simulink model "Buck_Due"  (R2020a)
settings: Solver=FixedStepAuto  StartTime=0.0  StopTime=10  FixedStep=T  RelTol=1e-3  EnableMultiTasking=on
undefined symbols (not defined in the file): C, Ki_IL, Kp_IL, Kp_Uc, L, rL, T, Ubat
libraries: arduinolib x12, simulink x8, powerlib_meascontrol x1
settings Model: SILPILModeSetting=veronly  ExtModeTrigDuration=2  Creator=Nguyen Tung  LastModifiedBy=Nguyen Tung
settings OptimizationCC: StrengthReduction=on  PassReuseOutputArgsAs=Individual arguments  ZeroExternalMemoryAtStartup=off  ZeroInternalMemoryAtStartup=off  MaxStackSize=64  OptimizeBlockOrder=speed  OptimizationPriority=Speed  OptimizationCustomize=off  MultiThreadedLoops=on  EfficientTunableParamExpr=on
settings DebuggingCC: ParameterTunabilityLossMsg=error
settings HardwareCC: ProdBitPerPointer=32  ProdBitPerSizeT=32  ProdBitPerPtrDiffT=32  ProdLargestAtomicInteger=Long  ProdLargestAtomicFloat=Double  ProdWordSize=32  ProdHWDeviceType=ARM Compatible->ARM Cortex
settings SFSimCC: MATLABDynamicMemAlloc=off
settings RTWCC: SystemTargetFile=ert.tlc  HardwareBoard=Arduino Due  TLCOptions=-aInlineSetEventsForThisBaseRateFcn=TLC_FALSE -aSuppressMultiTaskScheduler=TLC_FALSE -aRateBasedStepFcn=1  TemplateMakefile=ert_default_tmf  Toolchain=Arduino ARM  BuildConfiguration=Faster Runs
settings CodeAppCC: ForceParamTrailComments=on  IgnoreCustomStorageClasses=off  OperatorAnnotations=on  SimulinkDataObjDesc=on  SFDataObjDesc=on  InsertBlockDesc=on
settings ERTTargetCC: SupportContinuousTime=on  SupportVariableSizeSignals=on  ExtModeStaticAllocSize=10000

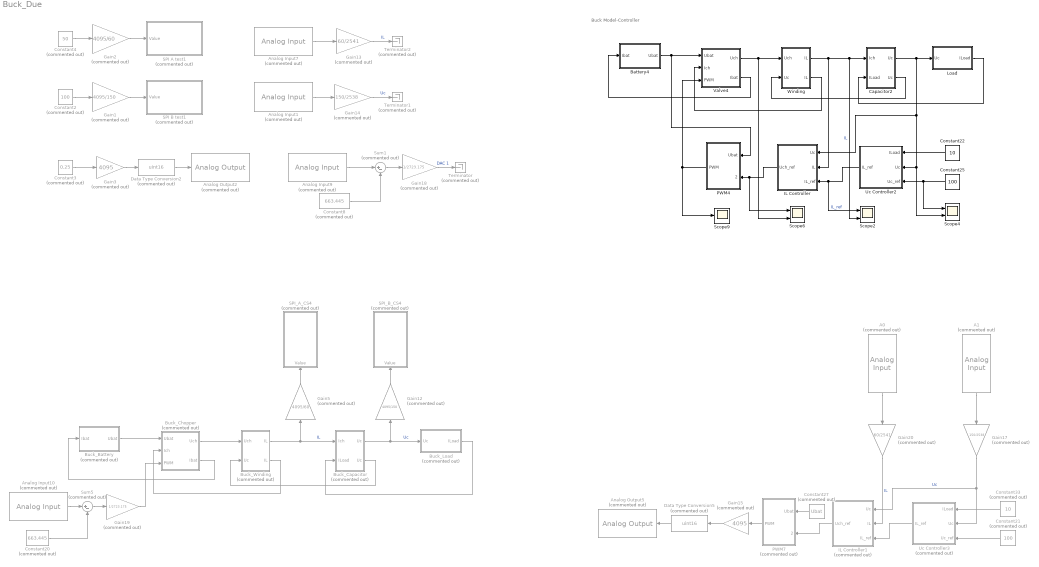
== system Buck_Due ==
  note: Buck Model-Controller
  A0 : arduinolib/Analog Input  Commented=on  pinNumber=0  ReadResultsOnly=off  ConversionTriggerSource=Software  ExternalTriggerType=uint32( 0 )  OutputDataType=uint16  EnableConversionCompleteNotify=off  EnableOuputStatus=off  SampleTime=T  blockPlatform=arduino
  A1 : arduinolib/Analog Input  Commented=on  pinNumber=1  ReadResultsOnly=off  ConversionTriggerSource=Software  ExternalTriggerType=uint32( 0 )  OutputDataType=uint16  EnableConversionCompleteNotify=off  EnableOuputStatus=off  SampleTime=T  blockPlatform=arduino
  Analog Input1 : arduinolib/Analog Input  Commented=on  pinNumber=1  ReadResultsOnly=off  ConversionTriggerSource=Software  ExternalTriggerType=uint32( 0 )  OutputDataType=uint16  EnableConversionCompleteNotify=off  EnableOuputStatus=off  SampleTime=T  blockPlatform=arduino
  Analog Input10 : arduinolib/Analog Input  Commented=on  pinNumber=1  ReadResultsOnly=off  ConversionTriggerSource=Software  ExternalTriggerType=uint32( 0 )  OutputDataType=uint16  EnableConversionCompleteNotify=off  EnableOuputStatus=off  SampleTime=T  blockPlatform=arduino
  Analog Input7 : arduinolib/Analog Input  Commented=on  pinNumber=0  ReadResultsOnly=off  ConversionTriggerSource=Software  ExternalTriggerType=uint32( 0 )  OutputDataType=uint16  EnableConversionCompleteNotify=off  EnableOuputStatus=off  SampleTime=T  blockPlatform=arduino
  Analog Input9 : arduinolib/Analog Input  Commented=on  pinNumber=1  ReadResultsOnly=off  ConversionTriggerSource=Software  ExternalTriggerType=uint32( 0 )  OutputDataType=uint16  EnableConversionCompleteNotify=off  EnableOuputStatus=off  SampleTime=T  blockPlatform=arduino
  Analog Output2 : arduinolib/Analog Output  Commented=on  DACpin=DAC1  blockPlatform=arduino
      settings: SourceProductBaseCode=ARDUINO
  Analog Output5 : arduinolib/Analog Output  Commented=on  DACpin=DAC1  blockPlatform=arduino
      settings: SourceProductBaseCode=ARDUINO
  Battery4 : Subsystem  AncestorBlock=simulink/REM/SE
      mask Display:
      | plot(0,0,100,100, 1.2*[50,57.68,60.77,63.08,64.97,66.58,68,69.26,70.4, 	71.42,72.36,78.28,80,78.28,72.36,71.42,70.4, 	69.26,68,66.58,64.97,63.08,60.77,57.68,50,42.32, 	39.23,36.92,35.03,33.42,32,30.74,29.6,28.58, 	27.64,21.72,20,21.72,27.64,28.58,29.6,30.74,32, 	33.42,35.03,36.92,39.23,42.32,50]-10, 1.2*[20,21,22,23,24,25,26,27,28,29,30,40,50,60,70,71,72, 	73,74,75,76,77,78,79,80,79,78,77,76,75,74,73,72, 	71,70,60,50,40,30,29,28,27,26,25,24,23,22,21,20]-10)
      | disp('ES')
  Buck_Battery : Subsystem  Commented=on  AncestorBlock=simulink/REM/SE
      mask Display:
      | plot(0,0,100,100, 1.2*[50,57.68,60.77,63.08,64.97,66.58,68,69.26,70.4, 	71.42,72.36,78.28,80,78.28,72.36,71.42,70.4, 	69.26,68,66.58,64.97,63.08,60.77,57.68,50,42.32, 	39.23,36.92,35.03,33.42,32,30.74,29.6,28.58, 	27.64,21.72,20,21.72,27.64,28.58,29.6,30.74,32, 	33.42,35.03,36.92,39.23,42.32,50]-10, 1.2*[20,21,22,23,24,25,26,27,28,29,30,40,50,60,70,71,72, 	73,74,75,76,77,78,79,80,79,78,77,76,75,74,73,72, 	71,70,60,50,40,30,29,28,27,26,25,24,23,22,21,20]-10)
      | disp('ES')
  Buck_Capacitor : Subsystem  Commented=on  AncestorBlock=simulink/REM/EA  mask(CM){}
      mask Display: plot(0,0,100,100,[10,10,90,90,10],[90,10,10,90,90], [10,90],[10,90])
  Buck_Chopper : Subsystem  Commented=on  AncestorBlock=simulink/REM/EC Elec  mask(Hacheur){}
      mask Display: plot(0,0,100,100,[10,10,90,90,10],[90,10,10,90,90])
  Buck_Load : Subsystem  Commented=on  AncestorBlock=simulink/REM/SE
      mask Display:
      | plot(0,0,100,100, 1.2*[50,57.68,60.77,63.08,64.97,66.58,68,69.26,70.4, 	71.42,72.36,78.28,80,78.28,72.36,71.42,70.4, 	69.26,68,66.58,64.97,63.08,60.77,57.68,50,42.32, 	39.23,36.92,35.03,33.42,32,30.74,29.6,28.58, 	27.64,21.72,20,21.72,27.64,28.58,29.6,30.74,32, 	33.42,35.03,36.92,39.23,42.32,50]-10, 1.2*[20,21,22,23,24,25,26,27,28,29,30,40,50,60,70,71,72, 	73,74,75,76,77,78,79,80,79,78,77,76,75,74,73,72, 	71,70,60,50,40,30,29,28,27,26,25,24,23,22,21,20]-10)
      | disp('MS')
  Buck_Winding : Subsystem  Commented=on  AncestorBlock=simulink/REM/EA  mask(CM){}
      mask Display: plot(0,0,100,100,[10,10,90,90,10],[90,10,10,90,90], [10,90],[10,90])
  Capacitor2 : Subsystem  AncestorBlock=simulink/REM/EA  mask(CM){}
      mask Display: plot(0,0,100,100,[10,10,90,90,10],[90,10,10,90,90], [10,90],[10,90])
  Constant2 : Constant  Commented=on  Value=100
  Constant20 : Constant  Commented=on  Value=663.445
  Constant21 : Constant  Commented=on  Value=100
  Constant22 : Constant  Value=10
  Constant25 : Constant  Value=100  SampleTime=T
  Constant27 : Constant  Commented=on  Value=Ubat
  Constant3 : Constant  Commented=on  Value=0.25
  Constant33 : Constant  Commented=on  Value=10
  Constant4 : Constant  Commented=on  Value=50
  Constant8 : Constant  Commented=on  Value=663.445
  Data Type Conversion2 : DataTypeConversion  Commented=on  OutDataTypeStr=uint16  RndMeth=Nearest
  Data Type Conversion5 : DataTypeConversion  Commented=on  OutDataTypeStr=uint16  RndMeth=Nearest
  Gain1 : Gain  Commented=on  Gain=4095/150
  Gain12 : Gain  Commented=on  Gain=4095/150
  Gain13 : Gain  Commented=on  Gain=60/2541
  Gain14 : Gain  Commented=on  Gain=150/2538
  Gain15 : Gain  Commented=on  Gain=4095
  Gain17 : Gain  Commented=on  Gain=150/2538
  Gain18 : Gain  Commented=on  Gain=1/2723.175
  Gain19 : Gain  Commented=on  Gain=1/2723.175
  Gain2 : Gain  Commented=on  Gain=4095/60
  Gain20 : Gain  Commented=on  Gain=60/2541
  Gain3 : Gain  Commented=on  Gain=4095
  Gain5 : Gain  Commented=on  Gain=4095/60
  IL Controller : Subsystem  AncestorBlock=simulink/SMC/Asservissement Correcteur IP
      mask Display: plot(0,0,100,100, [10,30,90,70,10,90],[90,10,10,90,90,10])
  IL Controller1 : Subsystem  Commented=on  AncestorBlock=simulink/SMC/Asservissement Correcteur IP
      mask Display: plot(0,0,100,100, [10,30,90,70,10,90],[90,10,10,90,90,10])
  Load : Subsystem  AncestorBlock=simulink/REM/SE
      mask Display:
      | plot(0,0,100,100, 1.2*[50,57.68,60.77,63.08,64.97,66.58,68,69.26,70.4, 	71.42,72.36,78.28,80,78.28,72.36,71.42,70.4, 	69.26,68,66.58,64.97,63.08,60.77,57.68,50,42.32, 	39.23,36.92,35.03,33.42,32,30.74,29.6,28.58, 	27.64,21.72,20,21.72,27.64,28.58,29.6,30.74,32, 	33.42,35.03,36.92,39.23,42.32,50]-10, 1.2*[20,21,22,23,24,25,26,27,28,29,30,40,50,60,70,71,72, 	73,74,75,76,77,78,79,80,79,78,77,76,75,74,73,72, 	71,70,60,50,40,30,29,28,27,26,25,24,23,22,21,20]-10)
      | disp('MS')
  PWM4 : Subsystem  AncestorBlock=simulink/SMC/Inversion EC avec mesure
      mask Display: plot(0,0,100,100,[10,30,90,70,10],[90,10,10,90,90])
  PWM7 : Subsystem  Commented=on  AncestorBlock=simulink/SMC/Inversion EC avec mesure
      mask Display: plot(0,0,100,100,[10,30,90,70,10],[90,10,10,90,90])
  SPI A test1 : Subsystem  Commented=on
  SPI B test1 : Subsystem  Commented=on
  SPI_A_CS4 : Subsystem  Commented=on
  SPI_B_CS4 : Subsystem  Commented=on
  Scope2 : Scope  NumInputPorts=2
  Scope4 : Scope  NumInputPorts=2
  Scope6 : Scope  NumInputPorts=2
  Scope9 : Scope
  Sum1 : Sum  Commented=on  Inputs=|+-
  Sum5 : Sum  Commented=on  Inputs=|+-
  Terminator : Terminator  Commented=on
  Terminator1 : Terminator  Commented=on
  Terminator2 : Terminator  Commented=on
  Uc Controller2 : Subsystem  AncestorBlock=simulink/SMC/Asservissement Correcteur IP
      mask Display: plot(0,0,100,100, [10,30,90,70,10,90],[90,10,10,90,90,10])
  Uc Controller3 : Subsystem  Commented=on  AncestorBlock=simulink/SMC/Asservissement Correcteur IP
      mask Display: plot(0,0,100,100, [10,30,90,70,10,90],[90,10,10,90,90,10])
  Valve4 : Subsystem  AncestorBlock=simulink/REM/EC Elec  mask(Hacheur){}
      mask Display: plot(0,0,100,100,[10,10,90,90,10],[90,10,10,90,90])
  Winding : Subsystem  AncestorBlock=simulink/REM/EA  mask(CM){}
      mask Display: plot(0,0,100,100,[10,10,90,90,10],[90,10,10,90,90], [10,90],[10,90])
  wires:
  Constant3/1 -> Gain3/1
  Constant2/1 -> Gain1/1
  Gain1/1 -> SPI B test1/1(Value)
  Constant8/1 -> Sum1/2
  Gain14/1 -> Terminator1/1  "Uc"
  Analog Input1/1 -> Gain14/1
  Sum1/1 -> Gain18/1
  Gain2/1 -> SPI A test1/1(Value)
  Analog Input9/1 -> Sum1/1
  Gain18/1 -> Terminator/1  "DAC 1"
  Gain13/1 -> Terminator2/1  "IL"
  Constant4/1 -> Gain2/1
  Gain3/1 -> Data Type Conversion2/1
  Analog Input7/1 -> Gain13/1
  Data Type Conversion2/1 -> Analog Output2/1
  Valve4/2(Ibat) -> Battery4/1(Ibat)
  Capacitor2/2("Uc ") -> Winding/2(Uc)
  Constant25/1 -> Scope4/1, Uc Controller2/3(Uc_ref)
  Valve4/1(Uch) -> Scope6/2, Winding/1(Uch)
  Capacitor2/1(Uc) -> Load/1(Uc), IL Controller/1(Uc), Scope4/2, Uc Controller2/2(Uc)
  Constant22/1 -> Uc Controller2/1(ILoad)
  Battery4/1(Ubat) -> Valve4/1(Ubat), PWM4/1(Ubat)
  Winding/2("IL ") -> Valve4/2(Ich)
  Winding/1(IL) -> Scope2/2, Capacitor2/1(Ich), IL Controller/2(IL)  "IL"
  Uc Controller2/1(IL_ref) -> Scope2/1, IL Controller/3(IL_ref)  "IL_ref"
  IL Controller/1(Uch_ref) -> Scope6/1, PWM4/2(Uch_ref)
  Gain17/1 -> IL Controller1/1(Uc), Uc Controller3/2(Uc)  "Uc"
  PWM7/1(PWM) -> Gain15/1
  Constant33/1 -> Uc Controller3/1(ILoad)
  Data Type Conversion5/1 -> Analog Output5/1
  Constant21/1 -> Uc Controller3/3(Uc_ref)
  Gain15/1 -> Data Type Conversion5/1
  IL Controller1/1(Uch_ref) -> PWM7/2(Uch_ref)
  A1/1 -> Gain17/1
  Constant27/1 -> PWM7/1(Ubat)
  Uc Controller3/1(IL_ref) -> IL Controller1/3(IL_ref)
  Gain12/1 -> SPI_B_CS4/1(Value)
  Constant20/1 -> Sum5/2
  Gain19/1 -> Buck_Chopper/3(PWM)
  Buck_Load/1(ILoad) -> Buck_Capacitor/2(ILoad)
  Buck_Winding/1(IL) -> Buck_Capacitor/1(Ich), Gain5/1  "IL"
  Buck_Battery/1(Ubat) -> Buck_Chopper/1(Ubat)
  Buck_Capacitor/1(Uc) -> Buck_Load/1(Uc), Gain12/1  "Uc"
  Analog Input10/1 -> Sum5/1
  Buck_Chopper/1(Uch) -> Buck_Winding/1(Uch)
  Sum5/1 -> Gain19/1
  Buck_Capacitor/2("Uc ") -> Buck_Winding/2(Uc)
  Buck_Chopper/2(Ibat) -> Buck_Battery/1(Ibat)
  Buck_Winding/2("IL ") -> Buck_Chopper/2(Ich)
  Gain5/1 -> SPI_A_CS4/1(Value)
  A0/1 -> Gain20/1
  Gain20/1 -> IL Controller1/2(IL)  "IL"
  PWM4/1(PWM) -> Valve4/3(PWM), Scope9/1
  Load/1(ILoad) -> Capacitor2/2(ILoad)

== system Buck_Due/Battery4 ==
  Ibat : Inport
  Constant : Constant  Value=Ubat  SampleTime=T
  Terminator : Terminator
  Ubat : Outport  InitialOutput=0  VectorParamsAs1DForOutWhenUnconnected=off
  wires:
  Constant/1 -> Ubat/1
  Ibat/1 -> Terminator/1

== system Buck_Due/Buck_Battery ==
  Ibat : Inport
  Constant : Constant  Value=Ubat
  Terminator : Terminator
  Ubat : Outport  InitialOutput=0  VectorParamsAs1DForOutWhenUnconnected=off
  wires:
  Constant/1 -> Ubat/1
  Ibat/1 -> Terminator/1

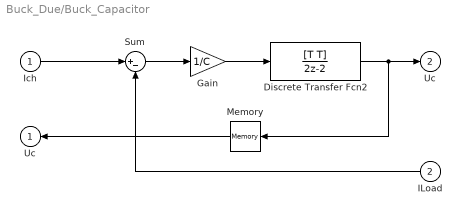
== system Buck_Due/Buck_Capacitor ==
  Ich : Inport
  ILoad : Inport  Port=2
  Discrete Transfer Fcn2 : DiscreteTransferFcn  Numerator=[T T]  Denominator=[2 -2]
  Gain : Gain  Gain=1/C
  Memory : Memory
  Sum : Sum  Inputs=|+-
  Uc : Outport  InitialOutput=0  VectorParamsAs1DForOutWhenUnconnected=off
  "Uc " : Outport  Port=2  InitialOutput=0  VectorParamsAs1DForOutWhenUnconnected=off
  wires:
  Ich/1 -> Sum/1
  Sum/1 -> Gain/1
  Gain/1 -> Discrete Transfer Fcn2/1
  Discrete Transfer Fcn2/1 -> "Uc "/1, Memory/1
  ILoad/1 -> Sum/2
  Memory/1 -> Uc/1

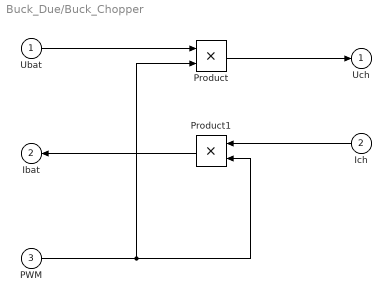
== system Buck_Due/Buck_Chopper ==
  Ubat : Inport
  Ich : Inport  Port=2
  PWM : Inport  Port=3
  Product : Product
  Product1 : Product
  Uch : Outport  InitialOutput=0  VectorParamsAs1DForOutWhenUnconnected=off
  Ibat : Outport  Port=2  InitialOutput=0  VectorParamsAs1DForOutWhenUnconnected=off
  wires:
  Product/1 -> Uch/1
  Ubat/1 -> Product/1
  PWM/1 -> Product1/2, Product/2
  Ich/1 -> Product1/1
  Product1/1 -> Ibat/1

== system Buck_Due/Buck_Load ==
  Uc : Inport
  Gain : Gain  Gain=1/10
  ILoad : Outport  InitialOutput=0  VectorParamsAs1DForOutWhenUnconnected=off
  wires:
  Uc/1 -> Gain/1
  Gain/1 -> ILoad/1

== system Buck_Due/Buck_Winding ==
  Uch : Inport
  Uc : Inport  Port=2
  Discrete Transfer Fcn : DiscreteTransferFcn  Numerator=[T T]  Denominator=[(2*L+rL*T) rL*T-2*L]
  Memory : Memory
  Sum : Sum  Inputs=|+-
  IL : Outport  InitialOutput=0  VectorParamsAs1DForOutWhenUnconnected=off
  "IL " : Outport  Port=2  InitialOutput=0  VectorParamsAs1DForOutWhenUnconnected=off
  wires:
  Uch/1 -> Sum/1
  Discrete Transfer Fcn/1 -> "IL "/1, Memory/1
  Sum/1 -> Discrete Transfer Fcn/1
  Uc/1 -> Sum/2
  Memory/1 -> IL/1

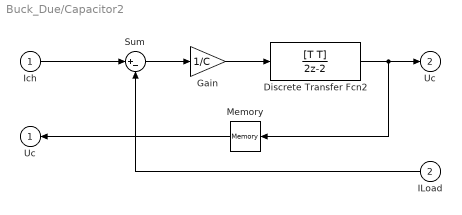
== system Buck_Due/Capacitor2 ==
  Ich : Inport
  ILoad : Inport  Port=2
  Discrete Transfer Fcn2 : DiscreteTransferFcn  Numerator=[T T]  Denominator=[2 -2]
  Gain : Gain  Gain=1/C
  Memory : Memory
  Sum : Sum  Inputs=|+-
  Uc : Outport  InitialOutput=0  VectorParamsAs1DForOutWhenUnconnected=off
  "Uc " : Outport  Port=2  InitialOutput=0  VectorParamsAs1DForOutWhenUnconnected=off
  wires:
  Ich/1 -> Sum/1
  Sum/1 -> Gain/1
  Gain/1 -> Discrete Transfer Fcn2/1
  Discrete Transfer Fcn2/1 -> "Uc "/1, Memory/1
  ILoad/1 -> Sum/2
  Memory/1 -> Uc/1

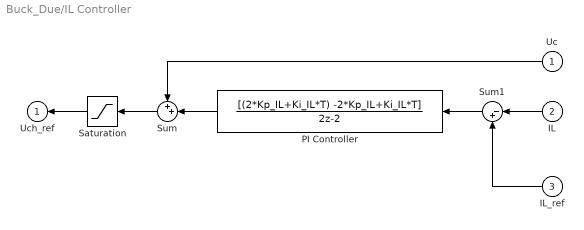
== system Buck_Due/IL Controller ==
  Uc : Inport
  IL : Inport  Port=2
  IL_ref : Inport  Port=3
  PI Controller : DiscreteTransferFcn  Numerator=[(2*Kp_IL+Ki_IL*T) -2*Kp_IL+Ki_IL*T]  Denominator=[2 -2]
  Saturation : Saturate  UpperLimit=Ubat  LowerLimit=0
  Sum : Sum  Inputs=++|
  Sum1 : Sum  Inputs=|-+
  Uch_ref : Outport  InitialOutput=0
  wires:
  Uc/1 -> Sum/1
  IL_ref/1 -> Sum1/2
  IL/1 -> Sum1/1
  Sum/1 -> Saturation/1
  Saturation/1 -> Uch_ref/1
  PI Controller/1 -> Sum/2
  Sum1/1 -> PI Controller/1

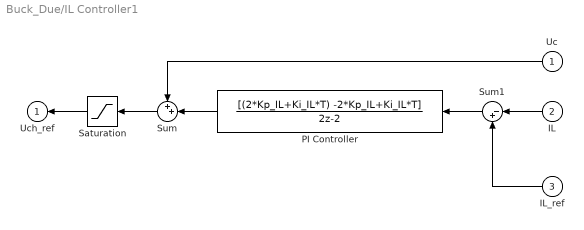
== system Buck_Due/IL Controller1 ==
  Uc : Inport
  IL : Inport  Port=2
  IL_ref : Inport  Port=3
  PI Controller : DiscreteTransferFcn  Numerator=[(2*Kp_IL+Ki_IL*T) -2*Kp_IL+Ki_IL*T]  Denominator=[2 -2]
  Saturation : Saturate  UpperLimit=Ubat  LowerLimit=0
  Sum : Sum  Inputs=++|
  Sum1 : Sum  Inputs=|-+
  Uch_ref : Outport  InitialOutput=0
  wires:
  Uc/1 -> Sum/1
  IL_ref/1 -> Sum1/2
  IL/1 -> Sum1/1
  Sum/1 -> Saturation/1
  Saturation/1 -> Uch_ref/1
  PI Controller/1 -> Sum/2
  Sum1/1 -> PI Controller/1

== system Buck_Due/Load ==
  Uc : Inport
  Gain : Gain  Gain=1/10
  ILoad : Outport  InitialOutput=0  VectorParamsAs1DForOutWhenUnconnected=off
  wires:
  Uc/1 -> Gain/1
  Gain/1 -> ILoad/1

== system Buck_Due/PWM4 ==
  Ubat : Inport
  Uch_ref : Inport  Port=2
  Divide : Product  Inputs=/*
  PWM Generator (DC-DC) : powerlib_meascontrol/Pulse & Signal Generators/PWM Generator (DC-DC)  Fsw=1000  Ts=T
  PWM : Outport
  wires:
  Divide/1 -> PWM Generator (DC-DC)/1
  Ubat/1 -> Divide/1
  Uch_ref/1 -> Divide/2
  PWM Generator (DC-DC)/1 -> PWM/1

== system Buck_Due/PWM7 ==
  Ubat : Inport
  Uch_ref : Inport  Port=2
  Divide : Product  Inputs=/*
  PWM : Outport
  wires:
  Divide/1 -> PWM/1
  Ubat/1 -> Divide/1
  Uch_ref/1 -> Divide/2

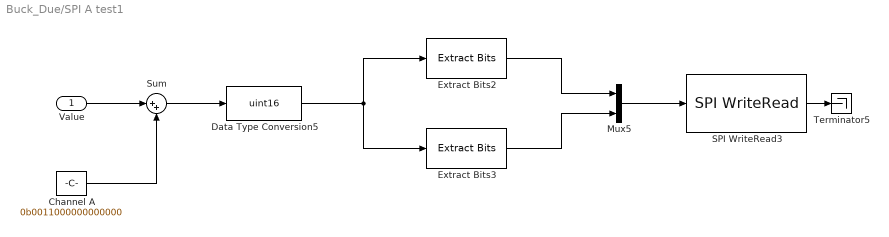
== system Buck_Due/SPI A test1 ==
  Value : Inport
  Channel A : Constant  Value=0b0011000000000000
  Data Type Conversion5 : DataTypeConversion  OutDataTypeStr=uint16  RndMeth=Nearest
  Extract Bits2 : simulink/Logic and Bit Operations/Extract Bits  bitsToExtract=Range starting with most significant bit  numBits=8  bitIdxRange=[0 7]  outScalingMode=Treat bit field as an integer
  Extract Bits3 : simulink/Logic and Bit Operations/Extract Bits  bitsToExtract=Range ending with least significant bit  numBits=8  bitIdxRange=[0 7]  outScalingMode=Treat bit field as an integer
  Mux5 : Mux  Inputs=2
  SPI WriteRead3 : arduinolib/SPI WriteRead  slaveSelectPin_=10  blockPlatform=arduino
      settings: SourceProductBaseCode=ARDUINO
  Sum : Sum  Inputs=|++
  Terminator5 : Terminator
  wires:
  Extract Bits3/1 -> Mux5/2
  Mux5/1 -> SPI WriteRead3/1
  Channel A/1 -> Sum/2
  Extract Bits2/1 -> Mux5/1
  Data Type Conversion5/1 -> Extract Bits2/1, Extract Bits3/1
  SPI WriteRead3/1 -> Terminator5/1
  Sum/1 -> Data Type Conversion5/1
  Value/1 -> Sum/1

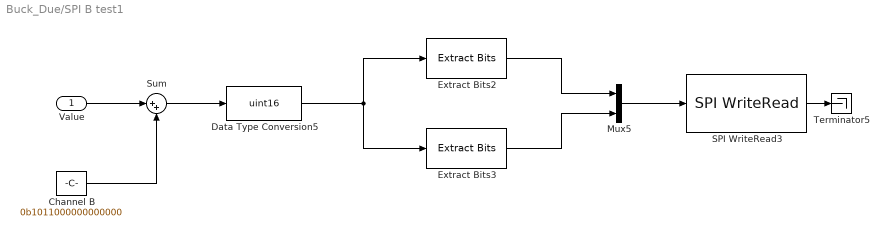
== system Buck_Due/SPI B test1 ==
  Value : Inport
  Channel B : Constant  Value=0b1011000000000000
  Data Type Conversion5 : DataTypeConversion  OutDataTypeStr=uint16  RndMeth=Nearest
  Extract Bits2 : simulink/Logic and Bit Operations/Extract Bits  bitsToExtract=Range starting with most significant bit  numBits=8  bitIdxRange=[0 7]  outScalingMode=Treat bit field as an integer
  Extract Bits3 : simulink/Logic and Bit Operations/Extract Bits  bitsToExtract=Range ending with least significant bit  numBits=8  bitIdxRange=[0 7]  outScalingMode=Treat bit field as an integer
  Mux5 : Mux  Inputs=2
  SPI WriteRead3 : arduinolib/SPI WriteRead  slaveSelectPin_=10  blockPlatform=arduino
      settings: SourceProductBaseCode=ARDUINO
  Sum : Sum  Inputs=|++
  Terminator5 : Terminator
  wires:
  Extract Bits3/1 -> Mux5/2
  Mux5/1 -> SPI WriteRead3/1
  Channel B/1 -> Sum/2
  Extract Bits2/1 -> Mux5/1
  Data Type Conversion5/1 -> Extract Bits2/1, Extract Bits3/1
  SPI WriteRead3/1 -> Terminator5/1
  Sum/1 -> Data Type Conversion5/1
  Value/1 -> Sum/1

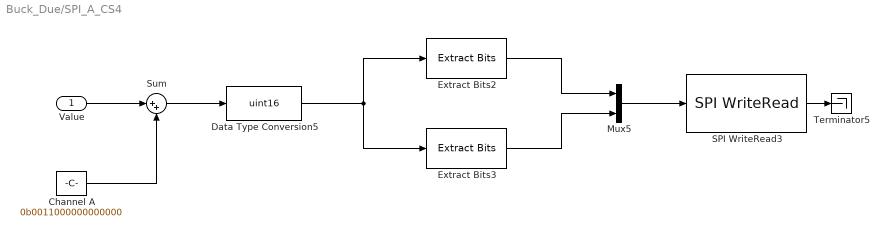
== system Buck_Due/SPI_A_CS4 ==
  Value : Inport
  Channel A : Constant  Value=0b0011000000000000
  Data Type Conversion5 : DataTypeConversion  OutDataTypeStr=uint16  RndMeth=Nearest
  Extract Bits2 : simulink/Logic and Bit Operations/Extract Bits  bitsToExtract=Range starting with most significant bit  numBits=8  bitIdxRange=[0 7]  outScalingMode=Treat bit field as an integer
  Extract Bits3 : simulink/Logic and Bit Operations/Extract Bits  bitsToExtract=Range ending with least significant bit  numBits=8  bitIdxRange=[0 7]  outScalingMode=Treat bit field as an integer
  Mux5 : Mux  Inputs=2
  SPI WriteRead3 : arduinolib/SPI WriteRead  slaveSelectPin_=4  blockPlatform=arduino
      settings: SourceProductBaseCode=ARDUINO
  Sum : Sum  Inputs=|++
  Terminator5 : Terminator
  wires:
  Extract Bits3/1 -> Mux5/2
  Mux5/1 -> SPI WriteRead3/1
  Channel A/1 -> Sum/2
  Extract Bits2/1 -> Mux5/1
  Data Type Conversion5/1 -> Extract Bits2/1, Extract Bits3/1
  SPI WriteRead3/1 -> Terminator5/1
  Sum/1 -> Data Type Conversion5/1
  Value/1 -> Sum/1

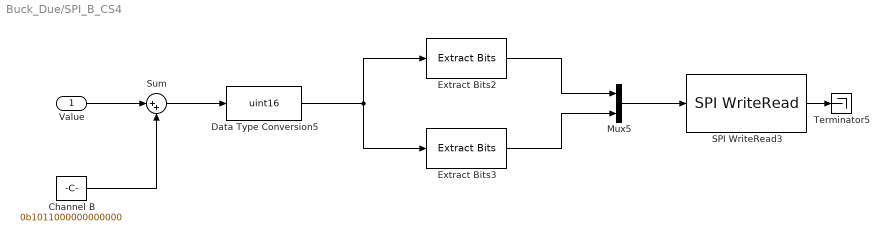
== system Buck_Due/SPI_B_CS4 ==
  Value : Inport
  Channel B : Constant  Value=0b1011000000000000
  Data Type Conversion5 : DataTypeConversion  OutDataTypeStr=uint16  RndMeth=Nearest
  Extract Bits2 : simulink/Logic and Bit Operations/Extract Bits  bitsToExtract=Range starting with most significant bit  numBits=8  bitIdxRange=[0 7]  outScalingMode=Treat bit field as an integer
  Extract Bits3 : simulink/Logic and Bit Operations/Extract Bits  bitsToExtract=Range ending with least significant bit  numBits=8  bitIdxRange=[0 7]  outScalingMode=Treat bit field as an integer
  Mux5 : Mux  Inputs=2
  SPI WriteRead3 : arduinolib/SPI WriteRead  slaveSelectPin_=4  blockPlatform=arduino
      settings: SourceProductBaseCode=ARDUINO
  Sum : Sum  Inputs=|++
  Terminator5 : Terminator
  wires:
  Extract Bits3/1 -> Mux5/2
  Mux5/1 -> SPI WriteRead3/1
  Channel B/1 -> Sum/2
  Extract Bits2/1 -> Mux5/1
  Data Type Conversion5/1 -> Extract Bits2/1, Extract Bits3/1
  SPI WriteRead3/1 -> Terminator5/1
  Sum/1 -> Data Type Conversion5/1
  Value/1 -> Sum/1

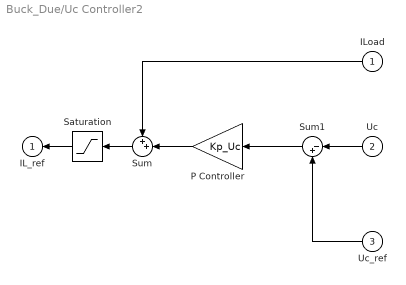
== system Buck_Due/Uc Controller2 ==
  ILoad : Inport
  Uc : Inport  Port=2
  Uc_ref : Inport  Port=3
  P Controller : Gain  Gain=Kp_Uc
  Saturation : Saturate  UpperLimit=60  LowerLimit=0
  Sum : Sum  Inputs=++|
  Sum1 : Sum  Inputs=|-+
  IL_ref : Outport  InitialOutput=0
  wires:
  Uc/1 -> Sum1/1
  Uc_ref/1 -> Sum1/2
  Sum1/1 -> P Controller/1
  P Controller/1 -> Sum/2
  ILoad/1 -> Sum/1
  Sum/1 -> Saturation/1
  Saturation/1 -> IL_ref/1

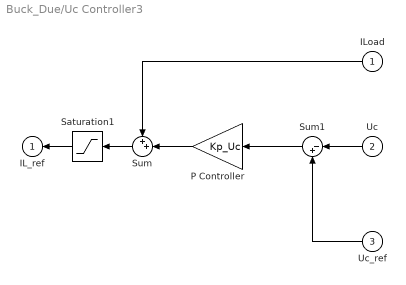
== system Buck_Due/Uc Controller3 ==
  ILoad : Inport
  Uc : Inport  Port=2
  Uc_ref : Inport  Port=3
  P Controller : Gain  Gain=Kp_Uc
  Saturation1 : Saturate  UpperLimit=60  LowerLimit=0
  Sum : Sum  Inputs=++|
  Sum1 : Sum  Inputs=|-+
  IL_ref : Outport  InitialOutput=0
  wires:
  Uc/1 -> Sum1/1
  Uc_ref/1 -> Sum1/2
  Sum1/1 -> P Controller/1
  P Controller/1 -> Sum/2
  ILoad/1 -> Sum/1
  Sum/1 -> Saturation1/1
  Saturation1/1 -> IL_ref/1

== system Buck_Due/Valve4 ==
  Ubat : Inport
  Ich : Inport  Port=2
  PWM : Inport  Port=3
  Product : Product
  Product1 : Product
  Uch : Outport  InitialOutput=0  VectorParamsAs1DForOutWhenUnconnected=off
  Ibat : Outport  Port=2  InitialOutput=0  VectorParamsAs1DForOutWhenUnconnected=off
  wires:
  Product/1 -> Uch/1
  Ubat/1 -> Product/1
  PWM/1 -> Product1/2, Product/2
  Ich/1 -> Product1/1
  Product1/1 -> Ibat/1

== system Buck_Due/Winding ==
  Uch : Inport
  Uc : Inport  Port=2
  Discrete Transfer Fcn : DiscreteTransferFcn  Numerator=[T T]  Denominator=[(2*L+rL*T) rL*T-2*L]
  Memory : Memory
  Sum : Sum  Inputs=|+-
  IL : Outport  InitialOutput=0  VectorParamsAs1DForOutWhenUnconnected=off
  "IL " : Outport  Port=2  InitialOutput=0  VectorParamsAs1DForOutWhenUnconnected=off
  wires:
  Uch/1 -> Sum/1
  Discrete Transfer Fcn/1 -> "IL "/1, Memory/1
  Sum/1 -> Discrete Transfer Fcn/1
  Uc/1 -> Sum/2
  Memory/1 -> IL/1
